simulink model "PDcontroller"  (R2017a)
settings: Solver=FixedStepAuto  StartTime=0.0  StopTime=50  FixedStep=0.05  RelTol=1e-3
settings Model: Creator=19101  LastModifiedBy=19101

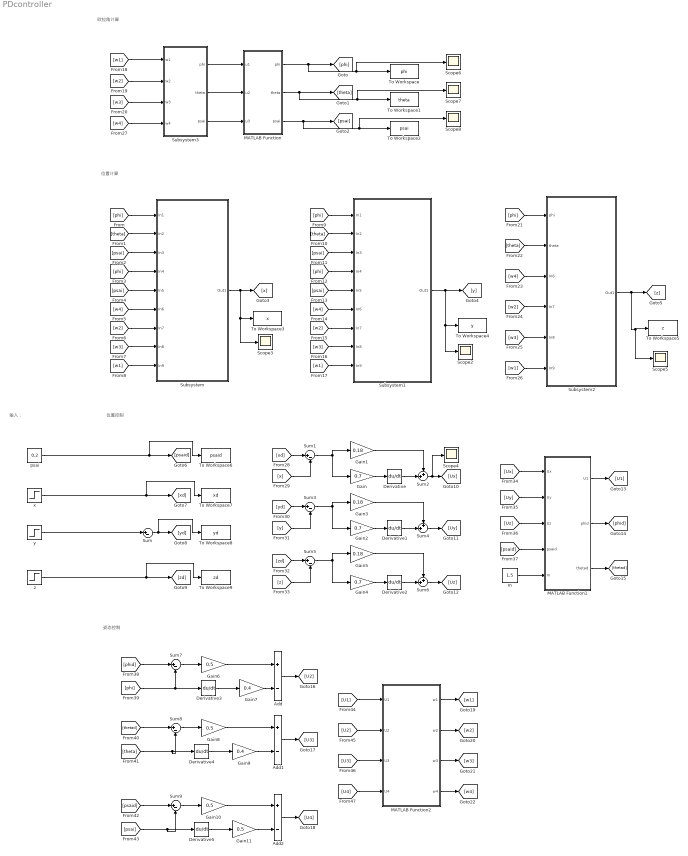
== system PDcontroller ==
  note: 位置计算
  note: 位置控制
  note: 输入：
  note: 姿态控制
  note: 欧拉角计算
  Add : Sum  Inputs=+-
  Add1 : Sum  Inputs=+-
  Add2 : Sum  Inputs=+-
  Derivative{,1..5} (6 alike) : Derivative
  Gain : Gain  Gain=0.7
  Gain1 : Gain  Gain=0.18
  Gain{6,8,10..11} (4 alike) : Gain  Gain=0.5
  Gain2 : Gain  Gain=0.7
  Gain3 : Gain  Gain=0.18
  Gain4 : Gain  Gain=0.7
  Gain5 : Gain  Gain=0.18
  Gain7 : Gain  Gain=0.4
  Gain9 : Gain  Gain=0.4
  MATLAB Function : MATLAB Function  TreatAsAtomicUnit=on
  MATLAB Function1 : MATLAB Function  TreatAsAtomicUnit=on
  MATLAB Function2 : MATLAB Function  TreatAsAtomicUnit=on
  Scope{2..8} (7 alike) : Scope
  Subsystem : Subsystem
  Subsystem1 : Subsystem
  Subsystem2 : Subsystem
  Subsystem3 : Subsystem
  Sum{,1,3,5,7..9} (7 alike) : Sum  Inputs=|+-
  Sum2 : Sum  Inputs=++|
  Sum4 : Sum  Inputs=++|
  Sum6 : Sum  Inputs=++|
  To Workspace : ToWorkspace  VariableName=phi  SampleTime=-1
  To Workspace1 : ToWorkspace  VariableName=theta  SampleTime=-1
  To Workspace2 : ToWorkspace  VariableName=psai  SampleTime=-1
  To Workspace3 : ToWorkspace  VariableName=x  SampleTime=-1
  To Workspace4 : ToWorkspace  VariableName=y  SampleTime=-1
  To Workspace5 : ToWorkspace  VariableName=z  SampleTime=-1
  To Workspace6 : ToWorkspace  VariableName=psaid  SampleTime=-1
  To Workspace7 : ToWorkspace  VariableName=xd  SampleTime=-1
  To Workspace8 : ToWorkspace  VariableName=yd  SampleTime=-1
  To Workspace9 : ToWorkspace  VariableName=zd  SampleTime=-1
  "m " : Constant  Value=1.5
  psai : Constant  Value=0.2
  x : Step  Time=20  Before=3  After=0  SampleTime=0
  y : Step  Time=10  After=3  SampleTime=0
  z : Step  Time=30  Before=3  After=0  SampleTime=0
  wires:
  [theta] -> Subsystem/2(In2)
  [phi] -> Subsystem/4(In4)
  [psai] -> Sum9/2, Derivative5/1
  Derivative1/1 -> Sum4/2
  [w3] -> Subsystem2/5(In8)
  Sum4/1 -> [Uy]
  Gain3/1 -> Sum4/1
  [phid] -> Sum7/1
  y/1 -> Sum/1
  Gain4/1 -> Derivative2/1
  Gain2/1 -> Derivative1/1
  [w2] -> Subsystem3/2(w2)
  Sum2/1 -> Scope4/1, [Ux]
  Gain9/1 -> Add1/2
  [zd] -> Sum5/1
  Gain5/1 -> Sum6/1
  Subsystem2/1(Out1) -> Scope5/1, To Workspace5/1, [z]
  Gain/1 -> Derivative/1
  [psaid] -> MATLAB Function1/4(psaid)
  [w4] -> Subsystem3/4(w4)
  [z] -> Sum5/2
  [theta] -> Subsystem1/2(In2)
  MATLAB Function1/2(phid) -> [phid]
  Sum6/1 -> [Uz]
  [w3] -> Subsystem1/8(In8)
  [theta] -> Subsystem2/2(theta)
  Subsystem3/3("psai ") -> MATLAB Function/3(u3)
  Subsystem3/2(theta) -> MATLAB Function/2(u2)
  [psai] -> Subsystem1/5(In5)
  Derivative3/1 -> Gain7/1
  Gain10/1 -> Add2/1
  [U3] -> MATLAB Function2/3(U3)
  [thetad] -> Sum8/1
  Gain11/1 -> Add2/2
  [xd] -> Sum1/1
  Gain6/1 -> Add/1
  Add/1 -> [U2]
  [Uy] -> MATLAB Function1/2(Uy)
  [w1] -> Subsystem2/6(In9)
  [U2] -> MATLAB Function2/2(U2)
  [x] -> Sum1/2
  [yd] -> Sum3/1
  MATLAB Function1/3(thetad) -> [thetad]
  [phi] -> Subsystem2/1(phi)
  "m "/1 -> MATLAB Function1/5(m)
  MATLAB Function1/1(U1) -> [U1]
  [U4] -> MATLAB Function2/4(U4)
  [phi] -> Subsystem/1(In1)
  [w1] -> Subsystem/9(In9)
  [y] -> Sum3/2
  Derivative/1 -> Sum2/2
  Gain7/1 -> Add/2
  Add2/1 -> [U4]
  psai/1 -> To Workspace6/1, [psaid]
  [theta] -> Sum8/2, Derivative4/1
  Sum5/1 -> Gain4/1, Gain5/1
  z/1 -> To Workspace9/1, [zd]
  Sum1/1 -> Gain/1, Gain1/1
  MATLAB Function2/4(w4) -> [w4]
  [psaid] -> Sum9/1
  Sum/1 -> To Workspace8/1, [yd]
  Subsystem3/1(phi) -> MATLAB Function/1(u1)
  x/1 -> To Workspace7/1, [xd]
  [Uz] -> MATLAB Function1/3(Uz)
  [w2] -> Subsystem2/4(In7)
  Gain1/1 -> Sum2/1
  MATLAB Function2/3(w3) -> [w3]
  Sum8/1 -> Gain8/1
  Add1/1 -> [U3]
  MATLAB Function/3(psai) -> To Workspace2/1, Scope8/1, [psai]
  MATLAB Function2/1(w1) -> [w1]
  [w4] -> Subsystem/6(In6)
  [w3] -> Subsystem3/3(w3)
  Derivative4/1 -> Gain9/1
  [Ux] -> MATLAB Function1/1(Ux)
  [w3] -> Subsystem/8(In8)
  [psai] -> Subsystem1/3(In3)
  [phi] -> Sum7/2, Derivative3/1
  Subsystem1/1(Out1) -> To Workspace4/1, Scope2/1, [y]
  [U1] -> MATLAB Function2/1(U1)
  Sum9/1 -> Gain10/1
  Derivative2/1 -> Sum6/2
  [phi] -> Subsystem1/4(In4)
  Gain8/1 -> Add1/1
  Subsystem/1(Out1) -> To Workspace3/1, Scope3/1, [x]
  MATLAB Function2/2(w2) -> [w2]
  [w4] -> Subsystem2/3(In6)
  [w1] -> Subsystem1/9(In9)
  [psai] -> Subsystem/3(In3)
  Sum3/1 -> Gain2/1, Gain3/1
  [w1] -> Subsystem3/1(w1)
  [phi] -> Subsystem1/1(In1)
  Derivative5/1 -> Gain11/1
  [w2] -> Subsystem/7(In7)
  [psai] -> Subsystem/5(In5)
  MATLAB Function/2(theta) -> To Workspace1/1, Scope7/1, [theta]
  Sum7/1 -> Gain6/1
  [w2] -> Subsystem1/7(In7)
  [w4] -> Subsystem1/6(In6)
  MATLAB Function/1(phi) -> Scope6/1, To Workspace/1, [phi]

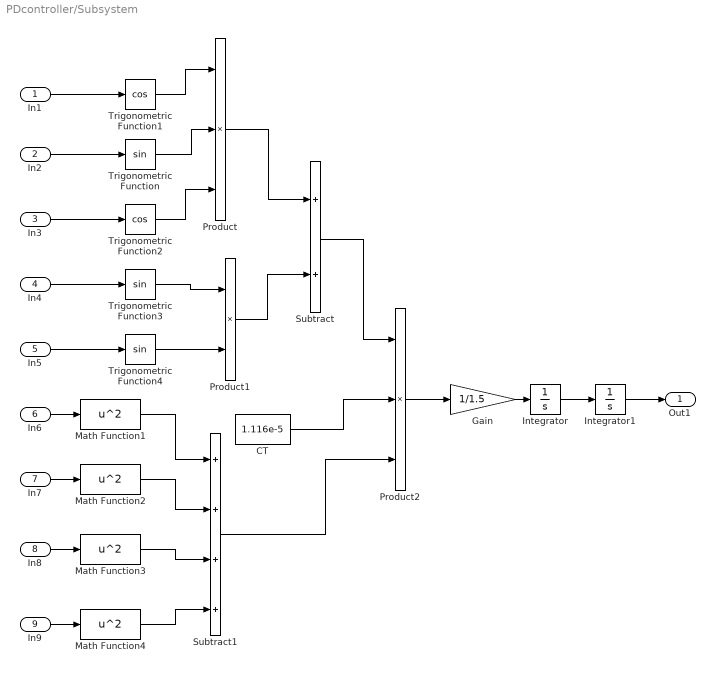
== system PDcontroller/Subsystem ==
  In1 : Inport
  In2 : Inport  Port=2
  In3 : Inport  Port=3
  In4 : Inport  Port=4
  In5 : Inport  Port=5
  In6 : Inport  Port=6
  In7 : Inport  Port=7
  In8 : Inport  Port=8
  In9 : Inport  Port=9
  CT : Constant  Value=1.116e-5
  Gain : Gain  Gain=1/1.5
  Integrator : Integrator
  Integrator1 : Integrator
  Math Function{1..4} (4 alike) : Math  Operator=square  SaturateOnIntegerOverflow=on
  Product : Product  Inputs=3
  Product1 : Product
  Product2 : Product  Inputs=3
  Subtract : Sum
  Subtract1 : Sum  Inputs=++++
  Trigonometric Function : Trigonometry
  Trigonometric Function1 : Trigonometry  Operator=cos
  Trigonometric Function2 : Trigonometry  Operator=cos
  Trigonometric Function3 : Trigonometry
  Trigonometric Function4 : Trigonometry
  Out1 : Outport
  wires:
  Trigonometric Function3/1 -> Product1/1
  Integrator1/1 -> Out1/1
  In3/1 -> Trigonometric Function2/1
  Subtract/1 -> Product2/1
  In4/1 -> Trigonometric Function3/1
  Integrator/1 -> Integrator1/1
  Product1/1 -> Subtract/2
  In1/1 -> Trigonometric Function1/1
  Trigonometric Function4/1 -> Product1/2
  Trigonometric Function/1 -> Product/2
  Product2/1 -> Gain/1
  CT/1 -> Product2/2
  In5/1 -> Trigonometric Function4/1
  In2/1 -> Trigonometric Function/1
  Trigonometric Function2/1 -> Product/3
  Gain/1 -> Integrator/1
  Product/1 -> Subtract/1
  Trigonometric Function1/1 -> Product/1
  In6/1 -> Math Function1/1
  In7/1 -> Math Function2/1
  In8/1 -> Math Function3/1
  In9/1 -> Math Function4/1
  Math Function1/1 -> Subtract1/1
  Math Function2/1 -> Subtract1/2
  Math Function3/1 -> Subtract1/3
  Math Function4/1 -> Subtract1/4
  Subtract1/1 -> Product2/3

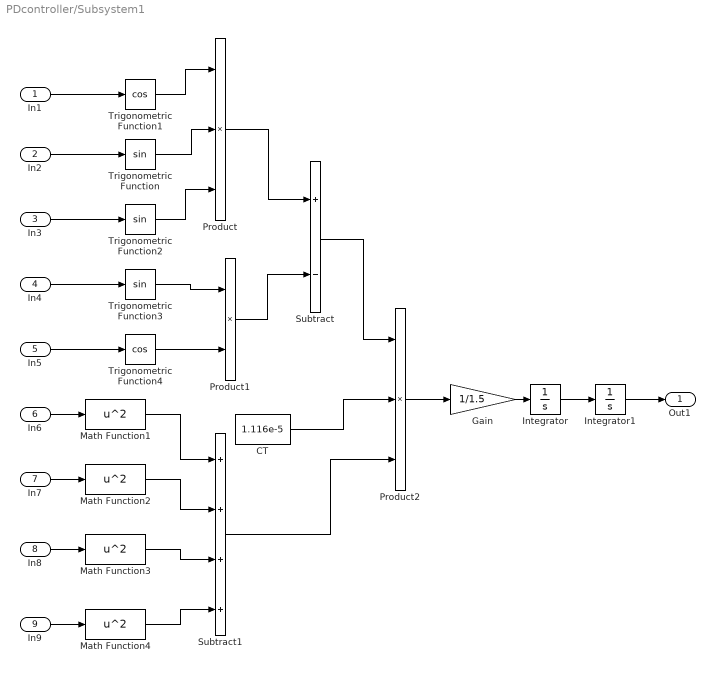
== system PDcontroller/Subsystem1 ==
  In1 : Inport
  In2 : Inport  Port=2
  In3 : Inport  Port=3
  In4 : Inport  Port=4
  In5 : Inport  Port=5
  In6 : Inport  Port=6
  In7 : Inport  Port=7
  In8 : Inport  Port=8
  In9 : Inport  Port=9
  CT : Constant  Value=1.116e-5
  Gain : Gain  Gain=1/1.5
  Integrator : Integrator
  Integrator1 : Integrator
  Math Function{1..4} (4 alike) : Math  Operator=square  SaturateOnIntegerOverflow=on
  Product : Product  Inputs=3
  Product1 : Product
  Product2 : Product  Inputs=3
  Subtract : Sum  Inputs=+-
  Subtract1 : Sum  Inputs=++++
  Trigonometric Function : Trigonometry
  Trigonometric Function1 : Trigonometry  Operator=cos
  Trigonometric Function2 : Trigonometry
  Trigonometric Function3 : Trigonometry
  Trigonometric Function4 : Trigonometry  Operator=cos
  Out1 : Outport
  wires:
  Trigonometric Function3/1 -> Product1/1
  Integrator1/1 -> Out1/1
  In3/1 -> Trigonometric Function2/1
  Subtract/1 -> Product2/1
  In4/1 -> Trigonometric Function3/1
  Integrator/1 -> Integrator1/1
  Product1/1 -> Subtract/2
  In1/1 -> Trigonometric Function1/1
  Trigonometric Function4/1 -> Product1/2
  Trigonometric Function/1 -> Product/2
  Product2/1 -> Gain/1
  CT/1 -> Product2/2
  In5/1 -> Trigonometric Function4/1
  In2/1 -> Trigonometric Function/1
  Trigonometric Function2/1 -> Product/3
  Gain/1 -> Integrator/1
  Product/1 -> Subtract/1
  Trigonometric Function1/1 -> Product/1
  Subtract1/1 -> Product2/3
  Math Function2/1 -> Subtract1/2
  Math Function1/1 -> Subtract1/1
  Math Function4/1 -> Subtract1/4
  Math Function3/1 -> Subtract1/3
  In6/1 -> Math Function1/1
  In7/1 -> Math Function2/1
  In8/1 -> Math Function3/1
  In9/1 -> Math Function4/1

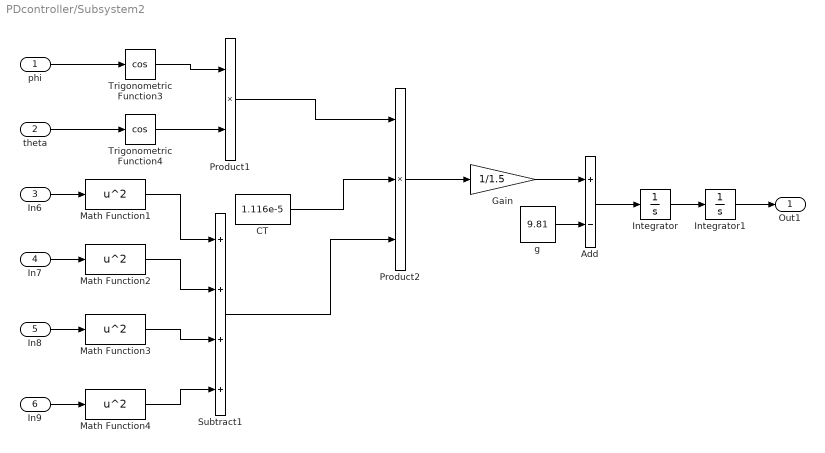
== system PDcontroller/Subsystem2 ==
  phi : Inport
  theta : Inport  Port=2
  In6 : Inport  Port=3
  In7 : Inport  Port=4
  In8 : Inport  Port=5
  In9 : Inport  Port=6
  Add : Sum  Inputs=+-
  CT : Constant  Value=1.116e-5
  Gain : Gain  Gain=1/1.5
  Integrator : Integrator
  Integrator1 : Integrator
  Math Function{1..4} (4 alike) : Math  Operator=square  SaturateOnIntegerOverflow=on
  Product1 : Product
  Product2 : Product  Inputs=3
  Subtract1 : Sum  Inputs=++++
  Trigonometric Function3 : Trigonometry  Operator=cos
  Trigonometric Function4 : Trigonometry  Operator=cos
  g : Constant  Value=9.81
  Out1 : Outport
  wires:
  Trigonometric Function3/1 -> Product1/1
  Integrator1/1 -> Out1/1
  phi/1 -> Trigonometric Function3/1
  Integrator/1 -> Integrator1/1
  Trigonometric Function4/1 -> Product1/2
  CT/1 -> Product2/2
  theta/1 -> Trigonometric Function4/1
  Product1/1 -> Product2/1
  g/1 -> Add/2
  Product2/1 -> Gain/1
  Gain/1 -> Add/1
  Add/1 -> Integrator/1
  Subtract1/1 -> Product2/3
  Math Function2/1 -> Subtract1/2
  Math Function1/1 -> Subtract1/1
  Math Function4/1 -> Subtract1/4
  Math Function3/1 -> Subtract1/3
  In6/1 -> Math Function1/1
  In7/1 -> Math Function2/1
  In8/1 -> Math Function3/1
  In9/1 -> Math Function4/1

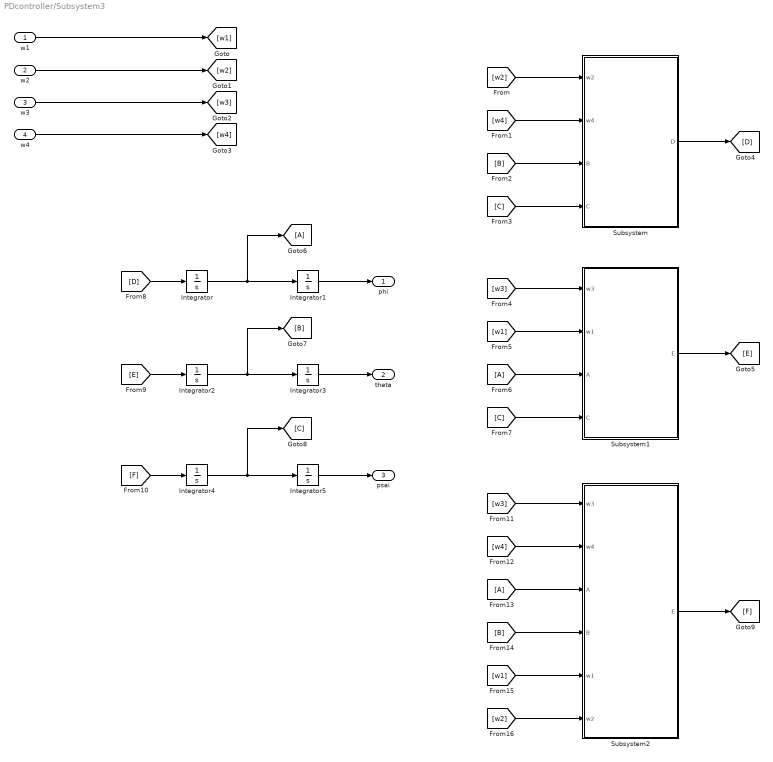
== system PDcontroller/Subsystem3 ==
  w1 : Inport
  w2 : Inport  Port=2
  w3 : Inport  Port=3
  w4 : Inport  Port=4
  Integrator{,1..5} (6 alike) : Integrator
  Subsystem : Subsystem
  Subsystem1 : Subsystem
  Subsystem2 : Subsystem
  phi : Outport
  theta : Outport  Port=2
  "psai " : Outport  Port=3
  wires:
  [w1] -> Subsystem2/5(w1)
  [w2] -> Subsystem2/6(w2)
  w4/1 -> [w4]
  w2/1 -> [w2]
  [w3] -> Subsystem1/1(w3)
  [A] -> Subsystem1/3(A)
  [w1] -> Subsystem1/2(w1)
  [C] -> Subsystem1/4(C)
  Subsystem1/1(E) -> [E]
  [B] -> Subsystem/3(B)
  [C] -> Subsystem/4(C)
  [w2] -> Subsystem/1(w2)
  [w4] -> Subsystem/2(w4)
  Subsystem/1(D) -> [D]
  w3/1 -> [w3]
  w1/1 -> [w1]
  Integrator/1 -> [A], Integrator1/1
  Integrator4/1 -> [C], Integrator5/1
  [F] -> Integrator4/1
  Integrator5/1 -> "psai "/1
  [E] -> Integrator2/1
  Integrator3/1 -> theta/1
  Integrator2/1 -> [B], Integrator3/1
  [D] -> Integrator/1
  Integrator1/1 -> phi/1
  [B] -> Subsystem2/4(B)
  Subsystem2/1(E) -> [F]
  [A] -> Subsystem2/3(A)
  [w4] -> Subsystem2/2(w4)
  [w3] -> Subsystem2/1(w3)

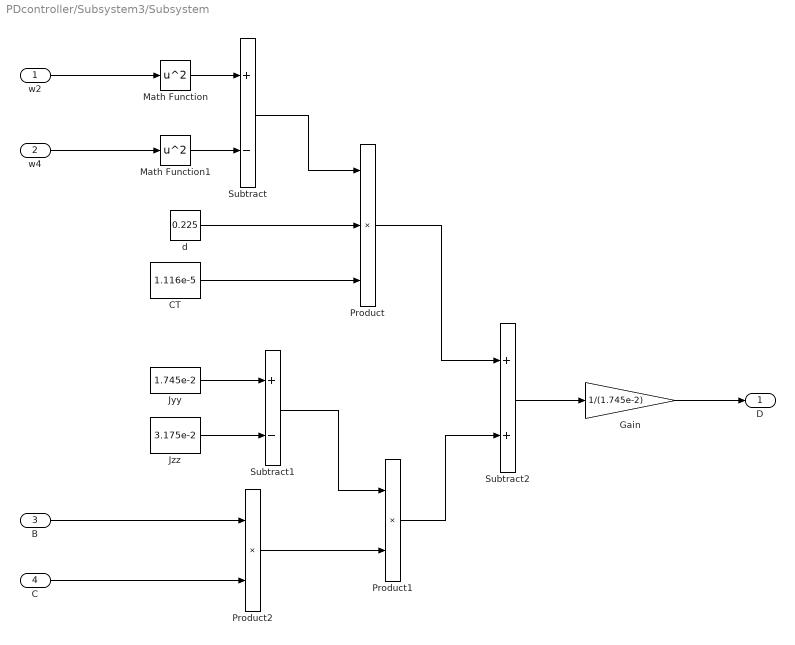
== system PDcontroller/Subsystem3/Subsystem ==
  w2 : Inport
  w4 : Inport  Port=2
  B : Inport  Port=3
  C : Inport  Port=4
  CT : Constant  Value=1.116e-5
  Gain : Gain  Gain=1/(1.745e-2)
  Jyy : Constant  Value=1.745e-2
  Jzz : Constant  Value=3.175e-2
  Math Function : Math  Operator=square  SaturateOnIntegerOverflow=on
  Math Function1 : Math  Operator=square  SaturateOnIntegerOverflow=on
  Product : Product  Inputs=3
  Product1 : Product
  Product2 : Product
  Subtract : Sum  Inputs=+-
  Subtract1 : Sum  Inputs=+-
  Subtract2 : Sum
  d : Constant  Value=0.225
  D : Outport
  wires:
  Gain/1 -> D/1
  Product2/1 -> Product1/2
  Subtract/1 -> Product/1
  w4/1 -> Math Function1/1
  Subtract2/1 -> Gain/1
  Math Function1/1 -> Subtract/2
  Jzz/1 -> Subtract1/2
  Product/1 -> Subtract2/1
  w2/1 -> Math Function/1
  B/1 -> Product2/1
  C/1 -> Product2/2
  Jyy/1 -> Subtract1/1
  d/1 -> Product/2
  CT/1 -> Product/3
  Product1/1 -> Subtract2/2
  Subtract1/1 -> Product1/1
  Math Function/1 -> Subtract/1

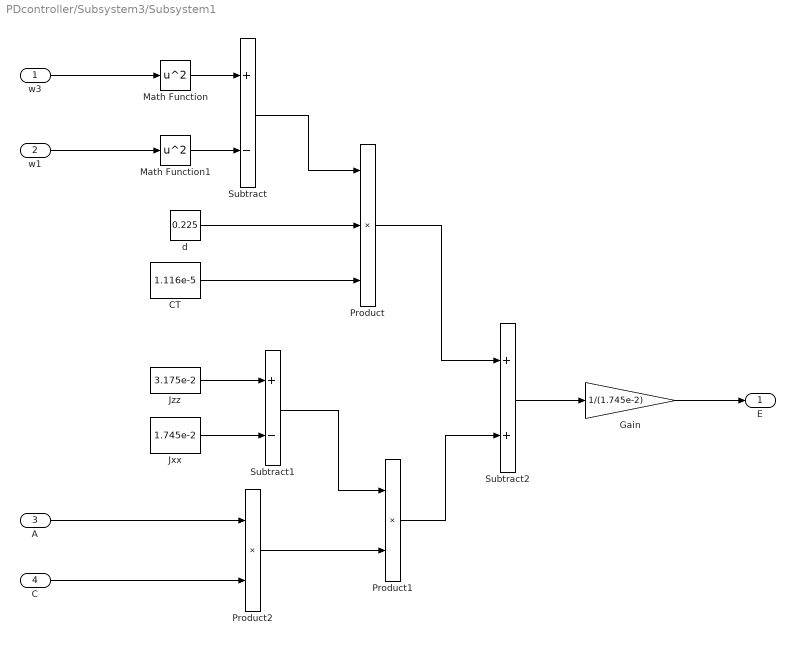
== system PDcontroller/Subsystem3/Subsystem1 ==
  w3 : Inport
  w1 : Inport  Port=2
  A : Inport  Port=3
  C : Inport  Port=4
  CT : Constant  Value=1.116e-5
  Gain : Gain  Gain=1/(1.745e-2)
  Jxx : Constant  Value=1.745e-2
  Jzz : Constant  Value=3.175e-2
  Math Function : Math  Operator=square  SaturateOnIntegerOverflow=on
  Math Function1 : Math  Operator=square  SaturateOnIntegerOverflow=on
  Product : Product  Inputs=3
  Product1 : Product
  Product2 : Product
  Subtract : Sum  Inputs=+-
  Subtract1 : Sum  Inputs=+-
  Subtract2 : Sum
  d : Constant  Value=0.225
  E : Outport
  wires:
  Gain/1 -> E/1
  Product2/1 -> Product1/2
  Subtract/1 -> Product/1
  w1/1 -> Math Function1/1
  Subtract2/1 -> Gain/1
  Math Function1/1 -> Subtract/2
  Jxx/1 -> Subtract1/2
  Product/1 -> Subtract2/1
  w3/1 -> Math Function/1
  A/1 -> Product2/1
  C/1 -> Product2/2
  Jzz/1 -> Subtract1/1
  d/1 -> Product/2
  CT/1 -> Product/3
  Product1/1 -> Subtract2/2
  Subtract1/1 -> Product1/1
  Math Function/1 -> Subtract/1

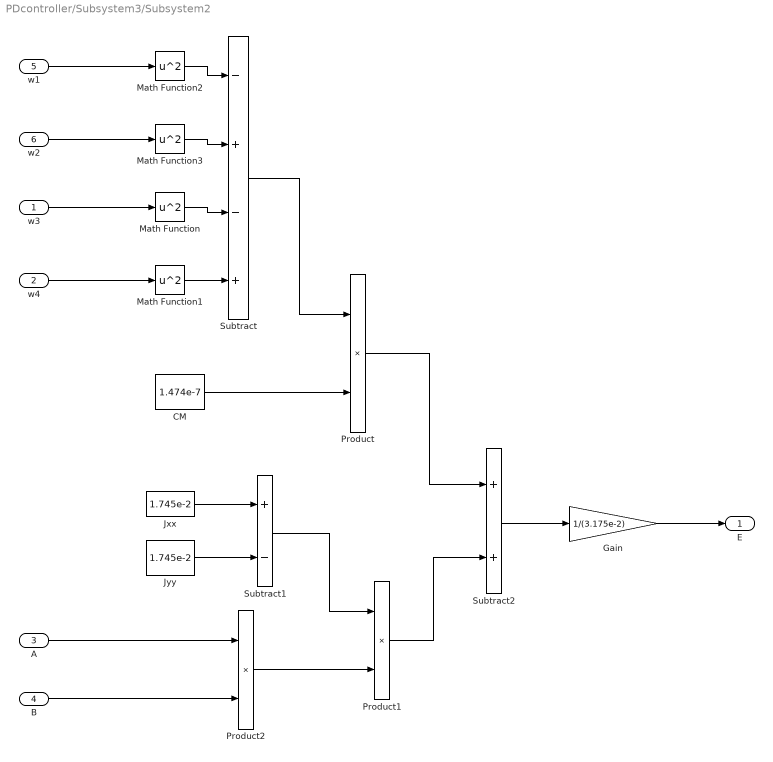
== system PDcontroller/Subsystem3/Subsystem2 ==
  w3 : Inport
  w4 : Inport  Port=2
  A : Inport  Port=3
  B : Inport  Port=4
  w1 : Inport  Port=5
  w2 : Inport  Port=6
  CM : Constant  Value=1.474e-7
  Gain : Gain  Gain=1/(3.175e-2)
  Jxx : Constant  Value=1.745e-2
  Jyy : Constant  Value=1.745e-2
  Math Function{,1..3} (4 alike) : Math  Operator=square  SaturateOnIntegerOverflow=on
  Product : Product
  Product1 : Product
  Product2 : Product
  Subtract : Sum  Inputs=-+-+
  Subtract1 : Sum  Inputs=+-
  Subtract2 : Sum
  E : Outport
  wires:
  Gain/1 -> E/1
  Product2/1 -> Product1/2
  Subtract/1 -> Product/1
  w4/1 -> Math Function1/1
  Subtract2/1 -> Gain/1
  Jyy/1 -> Subtract1/2
  Product/1 -> Subtract2/1
  w3/1 -> Math Function/1
  A/1 -> Product2/1
  B/1 -> Product2/2
  Jxx/1 -> Subtract1/1
  Product1/1 -> Subtract2/2
  Subtract1/1 -> Product1/1
  w1/1 -> Math Function2/1
  w2/1 -> Math Function3/1
  Math Function1/1 -> Subtract/4
  Math Function/1 -> Subtract/3
  Math Function3/1 -> Subtract/2
  Math Function2/1 -> Subtract/1
  CM/1 -> Product/2

== matlab function PDcontroller/MATLAB Function1 ==
  data: Ux input size=1; U1 output size=1; Uy input; Uz input; psaid input; m input; phid output; thetad output
function [U1,phid,thetad] = fcn(Ux,Uy,Uz,psaid,m)
    U1 = m*sqrt(Ux^2+Uy^2+(Uz+9.81)^2);
    phid = asin((Ux*sin(psaid)-Uy*cos(psaid))*m/U1);
    thetad = asin((Ux*m-U1*sin(psaid)*sin(phid))/(U1*cos(psaid)*cos(phid)));
end

== matlab function PDcontroller/MATLAB Function ==
  data: u1 input; phi output; u2 input; u3 input; theta output; psai output
function [phi,theta,psai] = fcn(u1,u2,u3)
phi=rem(u1,2*pi);
theta=rem(u2,2*pi);
psai=rem(u3,2*pi);
end

== matlab function PDcontroller/MATLAB Function2 ==
  data: U1 input; w1 output; U2 input; U3 input; U4 input; w2 output; w3 output; w4 output
function [w1,w2,w3,w4] = fcn(U1,U2,U3,U4)
    CT = 1.116e-5; dCT = 0.225*CT;
    matrixA = [CT,CT,CT,CT;0,CT,0,-CT;-CT,0,CT,0;-dCT,dCT,-dCT,dCT];
    w_2 = inv(matrixA)*[U1,U2,U3,U4]';
    w1 = sqrt(abs(w_2(1))); w2 = sqrt(abs(w_2(2)));
    w3 = sqrt(abs(w_2(3))); w4 = sqrt(abs(w_2(4)));
end
